simulink model "mophong"  (R2024a)
settings: Solver=VariableStepAuto  StartTime=0.0  StopTime=10.0  RelTol=1e-3
libraries: robotmobilelib x1, slpidlib x1
settings Model: Creator=dinhh  LastModifiedBy=dinhh

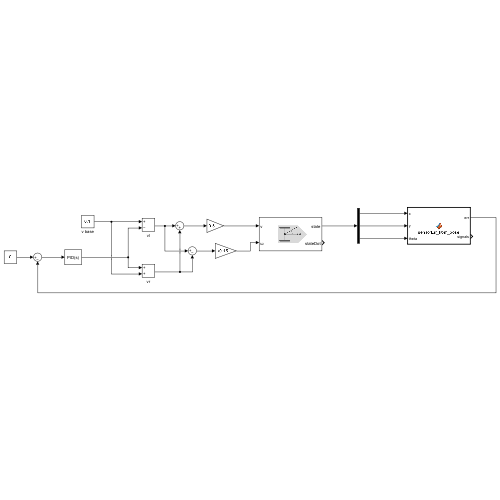
[thumbnail: Simulink's stored preview of the top-level diagram]
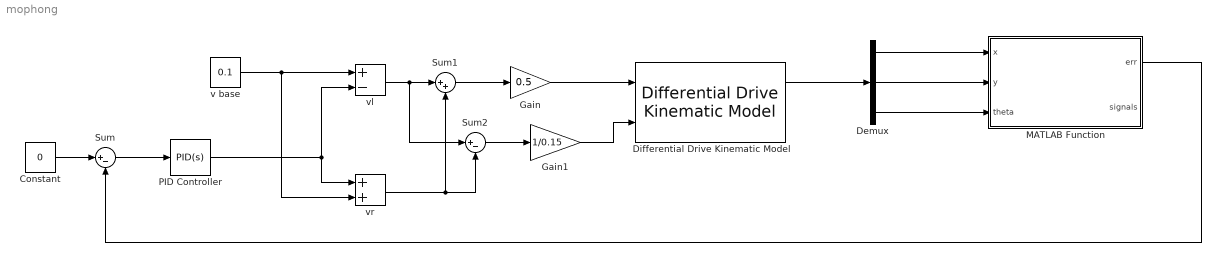
== system mophong ==
  Constant : Constant  Value=0
  Demux : Demux  Outputs=3
  Differential Drive Kinematic Model : robotmobilelib/Differential Drive Kinematic Model  VehicleInputs=Vehicle Speed & Heading Angular Velocity  WheelRadius=0.05  WheelSpeedRange=[-inf inf]  TrackWidth=0.15  InitialState=[3; 0; pi]  SimulateUsing=Code generation
  Gain : Gain  Gain=0.5
  Gain1 : Gain  Gain=1/0.15
  MATLAB Function : MATLAB Function  TreatAsAtomicUnit=on
  PID Controller : slpidlib/PID Controller  Controller=PID  Form=Parallel  TimeDomain=Continuous-time  UseExternalTs=off  SampleTime=-1  IntegratorMethod=Forward Euler  FilterMethod=Forward Euler  ControllerParametersSource=internal  P=1  I=1  UseKiTs=off  D=0  UseExternalDerivativeSource=off  N=100  UseFilter=on  TunerSelectOption=Transfer Function Based (PID Tuner App)  InitialConditionSource=internal  InitialConditionForIntegrator=0  InitialConditionForFilter=0  DifferentiatorICPrevScaledInput=0  ExternalReset=none  TrackingMode=off  Kt=1  LimitOutput=off  SatLimitsSource=internal  UpperSaturationLimit=inf  LowerSaturationLimit=-inf  LinearizeAsGain=on  AntiWindupMode=none  Kb=1  LimitIntegrator=off  UpperIntegratorSaturationLimit=inf  LowerIntegratorSaturationLimit=-inf  POutMin=[]  POutMax=[]  IOutMin=[]  IOutMax=[]  DOutMin=[]  DOutMax=[]  NOutMin=[]  NOutMax=[]  SumOutMin=[]  SumOutMax=[]  SaturationOutMin=[]  SaturationOutMax=[]  PParamMin=[]  PParamMax=[]  IParamMin=[]  IParamMax=[]  DParamMin=[]  DParamMax=[]  NParamMin=[]  NParamMax=[]  KbParamMin=[]  KbParamMax=[]  KtParamMin=[]  KtParamMax=[]  KbOutMin=[]  KbOutMax=[]  KtOutMin=[]  KtOutMax=[]  IntegratorOutMin=[]  IntegratorOutMax=[]  FilterOutMin=[]  FilterOutMax=[]  SumI1OutMin=[]  SumI1OutMax=[]  SumI2OutMin=[]  SumI2OutMax=[]  SumI3OutMin=[]  SumI3OutMax=[]  SumI4OutMin=[]  SumI4OutMax=[]  SumDOutMin=[]  SumDOutMax=[]  DifferentiatorOutMin=[]  DifferentiatorOutMax=[]  FilterDiffOutCoefMin=[]  FilterDiffOutCoefMax=[]  ReciprocalOutMin=[]  ReciprocalOutMax=[]  SumDenOutMin=[]  SumDenOutMax=[]  SumNumOutMin=[]  SumNumOutMax=[]  DivideOutMin=[]  DivideOutMax=[]  UdiffTsProdOutMin=[]  UdiffTsProdOutMax=[]  NTsProdOutMin=[]  NTsProdOutMax=[]  UintegralTsProdOutMin=[]  UintegralTsProdOutMax=[]  UngainTsProdOutMin=[]  UngainTsProdOutMax=[]  ClampingZeroOutDataTypeStr=Inherit: Inherit via back propagation  ClampingZeroOutMin=[]  ClampingZeroOutMax=[]  FilterDenConstantOutDataTypeStr=Inherit: Inherit via back propagation  FilterDenConstantOutMin=[]  FilterDenConstantOutMax=[]  PCopyOutDataTypeStr=Inherit: Inherit via back propagation  PCopyOutMin=[]  PCopyOutMax=[]  NCopyOutDataTypeStr=Inherit: Inherit via back propagation  NCopyOutMin=[]  NCopyOutMax=[]  IntegratorContinuousStateAttributes=''  IntegratorStateMustResolveToSignalObject=off  IntegratorRTWStateStorageClass=Auto  FilterContinuousStateAttributes=''  FilterStateMustResolveToSignalObject=off  FilterRTWStateStorageClass=Auto  ParallelPVariant=InternalParameters  IdealPVariant=Disabled  IVariant=InternalParameters  DVariant=InternalParameters  IntegratorVariant=Continuous  SatVariant=Disabled  AWVariant=Passthrough  PCopyVariant=Disabled  TRVariant=Disabled  FdbkBlocksVariant=Forward  IdealPFdbkVariant=Disabled  SatFdbkVariant=Disabled  DerivativeFilterVariant=ContFilter  NVariant=InternalParameters  NCopyVariant=Disabled  FilterICVariant=InternalICsFilter  IntegratorICVariant=InternalICs  ExternalResetVariant=Disabled  TRSumVariant=Passthrough  SumFdbkVariant=Disabled  SumVariant=Sum_PID  TsampFilterVariant=InternalTs  TsampNgainVariant=Passthrough  TsampIntegralVariant=Disabled_SignalSpec  ExternalSaturationOutDataTypeStr=Inherit: Same as second input  DerivativeSourceVariant=ErrorSignal
  Sum : Sum  Inputs=|+-
  Sum1 : Sum  Inputs=|++
  Sum2 : Sum  Inputs=|+-
  v base : Constant  Value=0.1
  vl : Sum  Inputs=+-
  vr : Sum
  wires:
  Constant/1 -> Sum/1
  MATLAB Function/1(err) -> Sum/2
  Sum/1 -> PID Controller/1
  PID Controller/1 -> vl/2, vr/1
  v base/1 -> vr/2, vl/1
  vl/1 -> Sum2/1, Sum1/1
  Sum1/1 -> Gain/1
  Gain/1 -> Differential Drive Kinematic Model/1
  vr/1 -> Sum1/2, Sum2/2
  Gain1/1 -> Differential Drive Kinematic Model/2
  Sum2/1 -> Gain1/1
  Demux/1 -> MATLAB Function/1(x)
  Demux/2 -> MATLAB Function/2(y)
  Demux/3 -> MATLAB Function/3(theta)
  Differential Drive Kinematic Model/1 -> Demux/1

== matlab function mophong/MATLAB Function ==
  data: err output; x input; signals output; y input; theta input
function [err, signals] = sensorErr_from_pose(x, y, theta)
% Inputs: x,y,theta (double scalars)
% Outputs:
%   err     : scalar error (double)
%   signals : 1x5 vector of 0/1 (double)

% ---- Track / parameters (hardcoded to match saban_nhap) ----
s = sqrt(2);
A = [3000, 0];
B = [500, 0];
C = [0, 500];
D = [500, 1000];
E = [1800 - 800*s, 1000];
F = [1800 - 400*s, 1800 - 400*s];
Hpt= [1800, 1500];
K  = [3000,1500];

R_arc2 = 800;
R_arc3 = 800;
trackWidth = 26;

% sensor geometry (same as your script)
d_sensor = 220;     % distance from robot center to sensor row
sensor_gap = 15;    % spacing between sensors
weights = [-2 -1 0 1 2];

% compute sensor positions (same formula as sensorPositions)
offsets = (-2:2)*sensor_gap;   % left->right
Xs = x + d_sensor*cos(theta) - offsets.*sin(theta);
Ys = y + d_sensor*sin(theta) + offsets.*cos(theta);

% check each sensor on track
signals = zeros(1,5);
for i=1:5
    signals(i) = checkPointOnTrack([Xs(i), Ys(i)], ...
                   A,B,C,D,E,F,Hpt,K,R_arc2, R_arc3, trackWidth);
end

% compute err
if sum(signals) > 0
    err = sum(weights .* signals) / sum(signals);
else
    % policy when lost line: return 0 (you can change to previous)
    err = 0;
end
end

% ----------------- helper functions (local) -----------------
function inside = checkPointOnTrack(P, A,B,C,D,E,F,Hpt,K,R_arc2,R_arc3,width)
% P is 1x2
tol = width/2 + 1e-6; % margin
x = P(1); y = P(2);
inside = false;

% segment AB (line)
if x >= min(A(1),B(1)) && x <= max(A(1),B(1))
    d = abs((B(2)-A(2))*(x-A(1)) - (B(1)-A(1))*(y-A(2))) / norm(B-A);
    if d <= tol, inside = true; return; end
end

% arc B->D (through C) using circleFrom3pts
[xc,yc,Rbd] = circleFrom3pts(B,C,D);
dR = abs(sqrt((x-xc)^2 + (y-yc)^2) - Rbd);
if dR <= tol
    if isAngleOnArc([x,y], xc,yc, B, D, false)  % false means not necessarily cw
        inside = true; return;
    end
end

% segment D->E (approx horizontal)
if x >= min(D(1),E(1)) && x <= max(D(1),E(1)) && abs(y - D(2)) <= tol
    inside = true; return;
end

% arc E->F (radius R_arc2)
[ok, Ox] = arcCenterSafe(E, F, R_arc2, false);
if ok
    dR2 = abs(norm([x,y]-Ox) - R_arc2);
    if dR2 <= tol
        if isAngleOnArc([x,y], Ox(1), Ox(2), E, F, false)
            inside = true; return;
        end
    end
end

% arc F->H (radius R_arc3) -- note: choose cw as in drawing (true)
[ok, Ox] = arcCenterSafe(F, Hpt, R_arc3, true);
if ok
    dR3 = abs(norm([x,y]-Ox) - R_arc3);
    if dR3 <= tol
        if isAngleOnArc([x,y], Ox(1), Ox(2), F, Hpt, true)
            inside = true; return;
        end
    end
end

% segment H->K
if x >= min(Hpt(1),K(1)) && x <= max(Hpt(1),K(1)) && abs(y - Hpt(2)) <= tol
    inside = true; return;
end
end

function [xc,yc,R] = circleFrom3pts(p1,p2,p3)
A = 2*[p2(1)-p1(1), p2(2)-p1(2); p3(1)-p1(1), p3(2)-p1(2)];
Bv = [p2(1)^2-p1(1)^2+p2(2)^2-p1(2)^2; p3(1)^2-p1(1)^2+p3(2)^2-p1(2)^2];
center = (A\Bv)';
xc = center(1); yc = center(2);
R = sqrt((p1(1)-xc)^2 + (p1(2)-yc)^2);
end

function [ok,O] = arcCenterSafe(P1,P2,R,cw)
M = (P1+P2)/2;
halfChord = norm(P2-P1)/2;
if halfChord > R+1e-9
    ok=false; O=[NaN NaN]; return;
end
h = sqrt(max(0,R^2-halfChord^2));
v = (P2-P1)/norm(P2-P1);
n = [-v(2), v(1)];
if cw, O = M - h*n; else O = M + h*n; end
ok=true;
end

function onarc = isAngleOnArc(P, xc, yc, Pstart, Pend, cw)
% returns true if angle(P) is within arc span from Pstart to Pend
angP = atan2(P(2)-yc, P(1)-xc);
ang1 = atan2(Pstart(2)-yc, Pstart(1)-xc);
ang2 = atan2(Pend(2)-yc, Pend(1)-xc);
if cw
    if ang2 > ang1, ang2 = ang2 - 2*pi; end
    angP = normalizeNear(angP, ang1);
    onarc = (angP <= ang1) && (angP >= ang2);
else
    if ang2 < ang1, ang2 = ang2 + 2*pi; end
    angP = normalizeNear(angP, ang1);
    onarc = (angP >= ang1) && (angP <= ang2);
end
end

function ang = normalizeNear(ang, ref)
while ang-ref > pi, ang = ang - 2*pi; end
while ang-ref < -pi, ang = ang + 2*pi; end
end
